simulink model "Tutorial4_RateAdaptive"  (R2020a)
settings: Solver=FixedStepAuto  StartTime=0.0  StopTime=10.0  FixedStep=1e-3  RelTol=1e-3  EnableMultiTasking=on
libraries: frdmk64flib x1
settings Model: ExtModeTrigDuration=5  Creator=haque  LastModifiedBy=haque
settings OptimizationCC: EnhancedBackFolding=on  PassReuseOutputArgsAs=Individual arguments  ZeroExternalMemoryAtStartup=off  ZeroInternalMemoryAtStartup=off  MaxStackSize=64  OptimizeBlockOrder=speed  DifferentSizesBufferReuse=on  OptimizationCustomize=off  EfficientTunableParamExpr=on
settings DebuggingCC: ParameterTunabilityLossMsg=error
settings HardwareCC: ProdBitPerPointer=32  ProdBitPerSizeT=32  ProdBitPerPtrDiffT=32  ProdLargestAtomicInteger=Long  ProdLargestAtomicFloat=Double  ProdWordSize=32  ProdHWDeviceType=ARM Compatible->ARM Cortex
settings SFSimCC: MATLABDynamicMemAlloc=off
settings RTWCC: SystemTargetFile=ert.tlc  HardwareBoard=NXP FRDM-K64F  TemplateMakefile=ert_default_tmf  Toolchain=GNU Tools for ARM Embedded Processors
settings CodeAppCC: ForceParamTrailComments=on  IgnoreCustomStorageClasses=off  OperatorAnnotations=on  SimulinkDataObjDesc=on  SFDataObjDesc=on  InsertBlockDesc=on

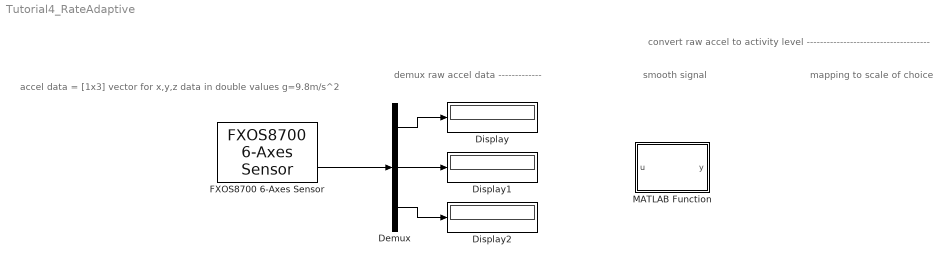
== system Tutorial4_RateAdaptive ==
  note: mapping to scale of choice
  note: smooth signal
  note: convert raw accel to activity level -------------------------------------
  note: demux raw accel data -------------
  note: accel data = [1x3] vector for x,y,z data in double values g=9.8m/s^2
  Demux : Demux  Outputs=3
  Display : Display
  Display1 : Display
  Display2 : Display
  FXOS8700 6-Axes Sensor : frdmk64flib/FXOS8700 6-Axes Sensor  Activesensor=Accelerometer and Magnetometer  ODR=800Hz  HybridODR=400Hz  Accelfullrange=-4g to +4g  SampleTime=-1
  MATLAB Function : MATLAB Function  TreatAsAtomicUnit=on
  wires:
  FXOS8700 6-Axes Sensor/2 -> Demux/1
  Demux/1 -> Display/1
  Demux/2 -> Display1/1
  Demux/3 -> Display2/1

== matlab function Tutorial4_RateAdaptive/MATLAB Function ==
  data: u input; y output
function y = SignalSmoothing(u)
%{ 
u = original signal --> plot (t, u(t))
y = smoothed signal --> plot (t, y(t))
%} 







y = u;


%{
EXAMPLE FROM MATLAB:
https://www.mathworks.com/help/signal/ug/signal-smoothing.html 

ORIGINAL SIGNAL:

load bostemp
days = (1:31*24)/24;
plot(days, tempC)
axis tight
ylabel("Temperature (\circC)")
xlabel("Time elapsed from Jan 1, 2011 (days)")
title("Logan Airport Dry Bulb Temperature (source: NOAA)")



SMOOTH SIGNAL VIA MOVING AVERAGE FILTER:
hoursPerDay = 24;
coeff24hMA = ones(1, hoursPerDay)/hoursPerDay;

avg24hTempC = filter(coeff24hMA, 1, tempC);
plot(days,[tempC avg24hTempC])
legend("Hourly Temp","24 Hour Average (delayed)","location","best")
ylabel("Temperature (\circC)")
xlabel("Time elapsed from Jan 1, 2011 (days)")
title("Logan Airport Dry Bulb Temperature (source: NOAA)")

%}
